simulink model "P2PHVDCMMC"  (R2024a)
settings: Solver=FixedStepDiscrete  StartTime=0.0  StopTime=10  RelTol=1e-3
PreLoadFcn:
  | % HVDCMMCInterconnectionParam
StartFcn:
  | tic
StopFcn:
  | toc
values from neighbouring files (symbols this model uses):
  C_PM = 1.758e-3    (= 0.001758)    [P2PHVDCMMCcode.m]
  Cg = 50e-9    (= 5e-08)    [P2PHVDCMMCcode.m]
  Fc = Fnom*3.37    (= 168.5)    [P2PHVDCMMCcode.m]
  Fnom = 50    [P2PHVDCMMCcode.m]
  Ki_Ireg = 6    [P2PHVDCMMCcode.m]
  Ki_Preg = 1.0    (= 1)    [P2PHVDCMMCcode.m]
  Ki_Qreg = 1.0    (= 1)    [P2PHVDCMMCcode.m]
  Ki_VDCreg = 100    [P2PHVDCMMCcode.m]
  Kp_Ireg = 0.6    [P2PHVDCMMCcode.m]
  Kp_Preg = 0.5/3    (= 0.166666666667)    [P2PHVDCMMCcode.m]
  Kp_Qreg = 0.5/3    (= 0.166666666667)    [P2PHVDCMMCcode.m]
  Kp_VDCreg = 4    [P2PHVDCMMCcode.m]
  L_cable = 15e-3    (= 0.015)    [P2PHVDCMMCcode.m]
  Larm = Larm_pu*(Zb_ac/(2*pi*Fnom))    [P2PHVDCMMCcode.m]
  Larm_pu = 0.15    [P2PHVDCMMCcode.m]
  Lff = Larm_pu/2    (= 0.075)    [P2PHVDCMMCcode.m]
  Limits_Ireg = [ 2.0  -2.0]    [P2PHVDCMMCcode.m]
  Limits_Preg = [ 1.2, 0.8 ]    [P2PHVDCMMCcode.m]
  Limits_Qreg = [ 0.25, -0.25 ]    [P2PHVDCMMCcode.m]
  Limits_VDCreg = [ 2.0  -2.0]    [P2PHVDCMMCcode.m]
  Lxfo = 0.12    [P2PHVDCMMCcode.m]
  N = 1    [P2PHVDCMMCcode.m]
  Nb_PM = 36    [P2PHVDCMMCcode.m]
  Pnom = 1000e6    (= 1000000000)    [P2PHVDCMMCcode.m]
  R_cable = 0.5    [P2PHVDCMMCcode.m]
  R_startup = 400    [P2PHVDCMMCcode.m]
  Rarm = Rarm_pu*Zb_ac    [P2PHVDCMMCcode.m]
  Rff = Rarm_pu/2    (= 0.00075)    [P2PHVDCMMCcode.m]
  Rg = 100    [P2PHVDCMMCcode.m]
  Rxfo = 0.003    [P2PHVDCMMCcode.m]
  Slope_Qref = 0.5    [P2PHVDCMMCcode.m]
  Slope_Vdc_ref = Vnom_dc/5    (= 128000)    [P2PHVDCMMCcode.m]
  Ts = Ts_Control    (= 4e-05)    [P2PHVDCMMCcode.m]
  Ts_Control = 40e-6    (= 4e-05)    [P2PHVDCMMCcode.m]
  Ts_Power = 20e-6    (= 2e-05)    [P2PHVDCMMCcode.m]
  Vnom_dc = 640e3    (= 640000)    [P2PHVDCMMCcode.m]
  Vnom_prim = 400e3    (= 400000)    [P2PHVDCMMCcode.m]
  Vnom_sec = 333e3    (= 333000)    [P2PHVDCMMCcode.m]
undefined symbols (not defined in the file or in its folder): DiscIntNeverNeededParam, Discrete, gcbh, HRM, Pcc, S, sps, sps_rtmsupport, spsMeanValueVariableFrequencyModel, spsPLL3phModel, SY3, Tfault
libraries: simulink x38, spsControlledVoltageSourceLib x30, DQsym_Lib x25, spsVoltageMeasurementLib x21, spsIdealSwitchLib x21, powerlib_extras x12, spsSecondOrderFilterLib x12, spsCurrentMeasurementLib x12, spsdq0toabcLib x9, spsMeanLib x8, spsMeanVariableFrequencyLib x8, spsabctodq0Lib x8
(part 2 of 8)

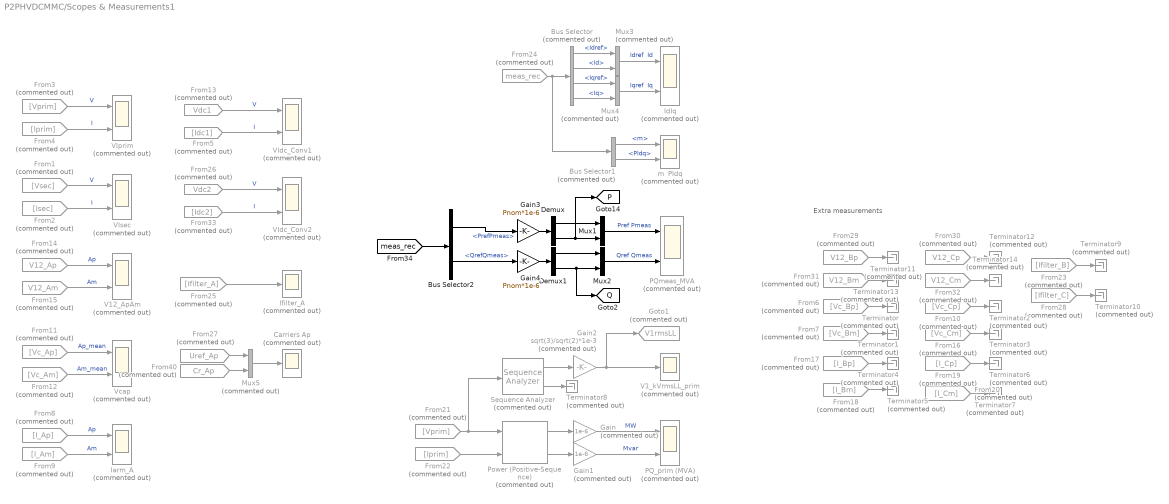
== system P2PHVDCMMC/Scopes & Measurements1 ==
  note: Extra measurements
  Bus Selector : BusSelector  Commented=on  OutputSignals=Idref,Id,Iqref,Iq
  Bus Selector1 : BusSelector  Commented=on  OutputSignals=m,PIdq
  Bus Selector2 : BusSelector  OutputSignals=PrefPmeas,QrefQmeas
  Carriers Ap : Scope  Commented=on
  Demux : Demux  Outputs=2
  Demux1 : Demux  Outputs=2
  From1 : From  Commented=on  GotoTag=Vsec  TagVisibility=global
  From10 : From  Commented=on  GotoTag=Vc_Cp
  From11 : From  Commented=on  GotoTag=Vc_Ap
  From12 : From  Commented=on  GotoTag=Vc_Am
  From13 : From  Commented=on  GotoTag=Vdc1  TagVisibility=global
  From14 : From  Commented=on  GotoTag=V12_Ap
  From15 : From  Commented=on  GotoTag=V12_Am
  From16 : From  Commented=on  GotoTag=Vc_Cm
  From17 : From  Commented=on  GotoTag=I_Bp
  From18 : From  Commented=on  GotoTag=I_Bm
  From19 : From  Commented=on  GotoTag=I_Cp
  From2 : From  Commented=on  GotoTag=Isec  TagVisibility=global
  From20 : From  Commented=on  GotoTag=I_Cm
  From21 : From  Commented=on  GotoTag=Vprim  TagVisibility=global
  From22 : From  Commented=on  GotoTag=Iprim  TagVisibility=global
  From23 : From  Commented=on  GotoTag=Ifilter_B
  From24 : From  Commented=on  GotoTag=meas_rec  TagVisibility=global
  From25 : From  Commented=on  GotoTag=Ifilter_A
  From26 : From  Commented=on  GotoTag=Vdc2  TagVisibility=global
  From27 : From  Commented=on  GotoTag=Uref_Ap  TagVisibility=global
  From28 : From  Commented=on  GotoTag=Ifilter_C
  From29 : From  Commented=on  GotoTag=V12_Bp
  From3 : From  Commented=on  GotoTag=Vprim  TagVisibility=global
  From30 : From  Commented=on  GotoTag=V12_Cp
  From31 : From  Commented=on  GotoTag=V12_Bm
  From32 : From  Commented=on  GotoTag=V12_Cm
  From33 : From  Commented=on  GotoTag=Idc2
  From4 : From  Commented=on  GotoTag=Iprim  TagVisibility=global
  From40 : From  Commented=on  GotoTag=Cr_Ap  TagVisibility=global
  From5 : From  Commented=on  GotoTag=Idc1  TagVisibility=global
  From6 : From  Commented=on  GotoTag=Vc_Bp
  From7 : From  Commented=on  GotoTag=Vc_Bm
  From8 : From  Commented=on  GotoTag=I_Ap
  From9 : From  Commented=on  GotoTag=I_Am
  Gain : Gain  Commented=on  Gain=1e-6
  Gain1 : Gain  Commented=on  Gain=1e-6
  Gain2 : Gain  Commented=on  Gain=sqrt(3)/sqrt(2)*1e-3
  Gain3 : Gain  Gain=Pnom*1e-6
  Gain4 : Gain  Gain=Pnom*1e-6
  Goto1 : Goto  Commented=on  GotoTag=V1rmsLL  TagVisibility=global
  Iarm_A : Scope  Commented=on  NumInputPorts=2
  IdIq : Scope  Commented=on  NumInputPorts=2
  Ifilter_A : Scope  Commented=on
  Mux1 : Mux  Inputs=2
  Mux2 : Mux  Inputs=2
  Mux3 : Mux  Commented=on  Inputs=2
  Mux4 : Mux  Commented=on  Inputs=2
  Mux5 : Mux  Commented=on  Inputs=2
  PQ_prim (MVA) : Scope  Commented=on  NumInputPorts=2
  PQmeas_MVA : Scope  Commented=on  NumInputPorts=2
  Power (Positive-Sequence) : spsPowerPositiveSequenceLib/Power (Positive-Sequence)  Commented=on  Freq=Fnom  Vinit=[0, 0]  Iinit=[0, 0]  Ts=Ts_Power
  Sequence Analyzer : spsSequenceAnalyzerLib/Sequence Analyzer  Commented=on  Freq=Fnom  n=1  seq=Positive  InInit=[1, 0]  Ts=Ts_Power
  Terminator{,1..14} (15 alike) : Terminator  Commented=on
  V12_ApAm : Scope  Commented=on  NumInputPorts=2
  V1_kVrmsLL_prim : Scope  Commented=on
  VIdc_Conv1 : Scope  Commented=on  NumInputPorts=2
  VIdc_Conv2 : Scope  Commented=on  NumInputPorts=2
  VIprim : Scope  Commented=on  NumInputPorts=2
  VIsec : Scope  Commented=on  NumInputPorts=2
  Vcap : Scope  Commented=on  NumInputPorts=2
  m  PIdq : Scope  Commented=on  NumInputPorts=2
  tag scope: P=global, Q=global
  wires:
  Mux5/1 -> Carriers Ap/1
  From40/1 -> Mux5/2
  From27/1 -> Mux5/1
  From12/1 -> Vcap/2  "Am_mean"
  From11/1 -> Vcap/1  "Ap_mean"
  From33/1 -> VIdc_Conv2/2  "I"
  From26/1 -> VIdc_Conv2/1  "V"
  Gain4/1 -> Demux1/1
  Gain3/1 -> Demux/1
  Mux2/1 -> PQmeas_MVA/2  "Qref Qmeas"
  Bus Selector2/2 -> Gain4/1  "<QrefQmeas>"
  Bus Selector2/1 -> Gain3/1  "<PrefPmeas>"
  Mux1/1 -> PQmeas_MVA/1  "Pref Pmeas"
  [meas_rec] -> Bus Selector2/1
  Gain2/1 -> V1_kVrmsLL_prim/1, Goto1/1
  Gain1/1 -> PQ_prim (MVA)/2  "Mvar"
  Gain/1 -> PQ_prim (MVA)/1  "MW"
  From32/1 -> Terminator14/1
  From31/1 -> Terminator13/1
  From30/1 -> Terminator12/1
  From29/1 -> Terminator11/1
  From28/1 -> Terminator10/1
  From23/1 -> Terminator9/1
  Sequence Analyzer/1 -> Gain2/1
  Power (Positive-Sequence)/2 -> Gain1/1
  Power (Positive-Sequence)/1 -> Gain/1
  Sequence Analyzer/2 -> Terminator8/1
  From22/1 -> Power (Positive-Sequence)/2
  From21/1 -> Power (Positive-Sequence)/1, Sequence Analyzer/1
  From5/1 -> VIdc_Conv1/2  "I"
  From13/1 -> VIdc_Conv1/1  "V"
  From25/1 -> Ifilter_A/1
  Bus Selector/4 -> Mux4/2  "<Iq>"
  Bus Selector/3 -> Mux4/1  "<Iqref>"
  Bus Selector/2 -> Mux3/2  "<Id>"
  Bus Selector/1 -> Mux3/1  "<Idref>"
  Mux4/1 -> IdIq/2  "Iqref  Iq"
  Mux3/1 -> IdIq/1  "Idref  Id"
  Bus Selector1/2 -> m  PIdq/2  "<PIdq>"
  Bus Selector1/1 -> m  PIdq/1  "<m>"
  From24/1 -> Bus Selector/1, Bus Selector1/1
  From20/1 -> Terminator7/1
  From19/1 -> Terminator6/1
  From18/1 -> Terminator5/1
  From17/1 -> Terminator4/1
  From9/1 -> Iarm_A/2  "Am"
  From8/1 -> Iarm_A/1  "Ap"
  From16/1 -> Terminator3/1
  From10/1 -> Terminator2/1
  From7/1 -> Terminator1/1
  From6/1 -> Terminator/1
  From15/1 -> V12_ApAm/2  "Am"
  From14/1 -> V12_ApAm/1  "Ap"
  From1/1 -> VIsec/1  "V"
  From2/1 -> VIsec/2  "I"
  From3/1 -> VIprim/1  "V"
  From4/1 -> VIprim/2  "I"
  Demux/1 -> Mux1/1
  Demux/2 -> [P], Mux1/2
  Demux1/1 -> Mux2/1
  Demux1/2 -> [Q], Mux2/2

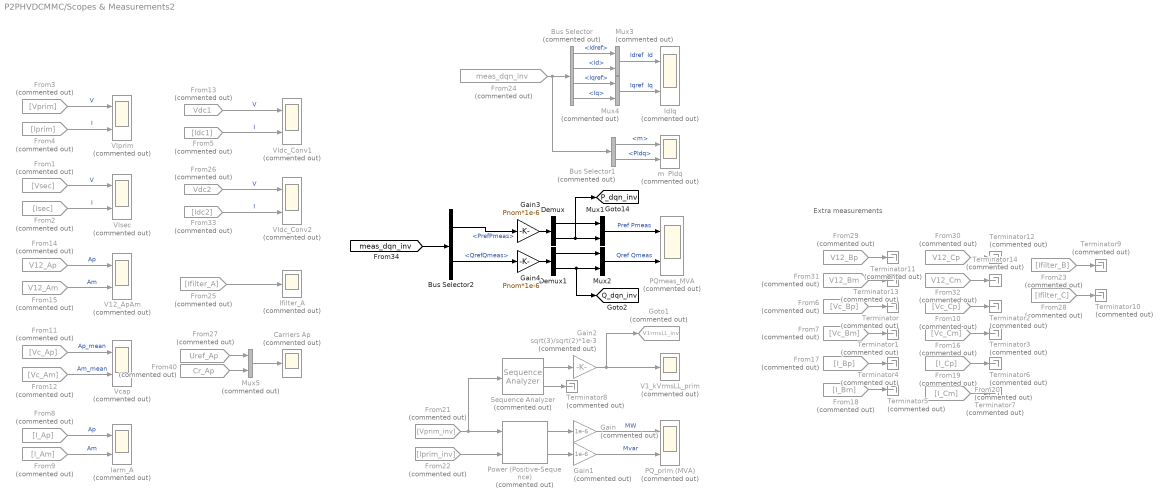
== system P2PHVDCMMC/Scopes & Measurements2 ==
  note: Extra measurements
  Bus Selector : BusSelector  Commented=on  OutputSignals=Idref,Id,Iqref,Iq
  Bus Selector1 : BusSelector  Commented=on  OutputSignals=m,PIdq
  Bus Selector2 : BusSelector  OutputSignals=PrefPmeas,QrefQmeas
  Carriers Ap : Scope  Commented=on
  Demux : Demux  Outputs=2
  Demux1 : Demux  Outputs=2
  From1 : From  Commented=on  GotoTag=Vsec  TagVisibility=global
  From10 : From  Commented=on  GotoTag=Vc_Cp
  From11 : From  Commented=on  GotoTag=Vc_Ap
  From12 : From  Commented=on  GotoTag=Vc_Am
  From13 : From  Commented=on  GotoTag=Vdc1  TagVisibility=global
  From14 : From  Commented=on  GotoTag=V12_Ap
  From15 : From  Commented=on  GotoTag=V12_Am
  From16 : From  Commented=on  GotoTag=Vc_Cm
  From17 : From  Commented=on  GotoTag=I_Bp
  From18 : From  Commented=on  GotoTag=I_Bm
  From19 : From  Commented=on  GotoTag=I_Cp
  From2 : From  Commented=on  GotoTag=Isec  TagVisibility=global
  From20 : From  Commented=on  GotoTag=I_Cm
  From21 : From  Commented=on  GotoTag=Vprim_inv  TagVisibility=global
  From22 : From  Commented=on  GotoTag=Iprim_inv  TagVisibility=global
  From23 : From  Commented=on  GotoTag=Ifilter_B
  From24 : From  Commented=on  GotoTag=meas_dqn_inv  TagVisibility=global
  From25 : From  Commented=on  GotoTag=Ifilter_A
  From26 : From  Commented=on  GotoTag=Vdc2  TagVisibility=global
  From27 : From  Commented=on  GotoTag=Uref_Ap  TagVisibility=global
  From28 : From  Commented=on  GotoTag=Ifilter_C
  From29 : From  Commented=on  GotoTag=V12_Bp
  From3 : From  Commented=on  GotoTag=Vprim  TagVisibility=global
  From30 : From  Commented=on  GotoTag=V12_Cp
  From31 : From  Commented=on  GotoTag=V12_Bm
  From32 : From  Commented=on  GotoTag=V12_Cm
  From33 : From  Commented=on  GotoTag=Idc2  TagVisibility=global
  From4 : From  Commented=on  GotoTag=Iprim  TagVisibility=global
  From40 : From  Commented=on  GotoTag=Cr_Ap  TagVisibility=global
  From5 : From  Commented=on  GotoTag=Idc1  TagVisibility=global
  From6 : From  Commented=on  GotoTag=Vc_Bp
  From7 : From  Commented=on  GotoTag=Vc_Bm
  From8 : From  Commented=on  GotoTag=I_Ap
  From9 : From  Commented=on  GotoTag=I_Am
  Gain : Gain  Commented=on  Gain=1e-6
  Gain1 : Gain  Commented=on  Gain=1e-6
  Gain2 : Gain  Commented=on  Gain=sqrt(3)/sqrt(2)*1e-3
  Gain3 : Gain  Gain=Pnom*1e-6
  Gain4 : Gain  Gain=Pnom*1e-6
  Goto1 : Goto  Commented=on  GotoTag=V1rmsLL_inv  TagVisibility=global
  Iarm_A : Scope  Commented=on  NumInputPorts=2
  IdIq : Scope  Commented=on  NumInputPorts=2
  Ifilter_A : Scope  Commented=on
  Mux1 : Mux  Inputs=2
  Mux2 : Mux  Inputs=2
  Mux3 : Mux  Commented=on  Inputs=2
  Mux4 : Mux  Commented=on  Inputs=2
  Mux5 : Mux  Commented=on  Inputs=2
  PQ_prim (MVA) : Scope  Commented=on  NumInputPorts=2
  PQmeas_MVA : Scope  Commented=on  NumInputPorts=2
  Power (Positive-Sequence) : spsPowerPositiveSequenceLib/Power (Positive-Sequence)  Commented=on  Freq=Fnom  Vinit=[0, 0]  Iinit=[0, 0]  Ts=Ts_Power
  Sequence Analyzer : spsSequenceAnalyzerLib/Sequence Analyzer  Commented=on  Freq=Fnom  n=1  seq=Positive  InInit=[1, 0]  Ts=Ts_Power
  Terminator{,1..14} (15 alike) : Terminator  Commented=on
  V12_ApAm : Scope  Commented=on  NumInputPorts=2
  V1_kVrmsLL_prim : Scope  Commented=on
  VIdc_Conv1 : Scope  Commented=on  NumInputPorts=2
  VIdc_Conv2 : Scope  Commented=on  NumInputPorts=2
  VIprim : Scope  Commented=on  NumInputPorts=2
  VIsec : Scope  Commented=on  NumInputPorts=2
  Vcap : Scope  Commented=on  NumInputPorts=2
  m  PIdq : Scope  Commented=on  NumInputPorts=2
  tag scope: P_dqn_inv=global, Q_dqn_inv=global
  wires:
  Demux1/2 -> Mux2/2, [Q_dqn_inv]
  Demux1/1 -> Mux2/1
  Demux/2 -> Mux1/2, [P_dqn_inv]
  Demux/1 -> Mux1/1
  From4/1 -> VIprim/2  "I"
  From3/1 -> VIprim/1  "V"
  From2/1 -> VIsec/2  "I"
  From1/1 -> VIsec/1  "V"
  From14/1 -> V12_ApAm/1  "Ap"
  From15/1 -> V12_ApAm/2  "Am"
  From6/1 -> Terminator/1
  From7/1 -> Terminator1/1
  From10/1 -> Terminator2/1
  From16/1 -> Terminator3/1
  From8/1 -> Iarm_A/1  "Ap"
  From9/1 -> Iarm_A/2  "Am"
  From17/1 -> Terminator4/1
  From18/1 -> Terminator5/1
  From19/1 -> Terminator6/1
  From20/1 -> Terminator7/1
  From24/1 -> Bus Selector1/1, Bus Selector/1
  Bus Selector1/1 -> m  PIdq/1  "<m>"
  Bus Selector1/2 -> m  PIdq/2  "<PIdq>"
  Mux3/1 -> IdIq/1  "Idref  Id"
  Mux4/1 -> IdIq/2  "Iqref  Iq"
  Bus Selector/1 -> Mux3/1  "<Idref>"
  Bus Selector/2 -> Mux3/2  "<Id>"
  Bus Selector/3 -> Mux4/1  "<Iqref>"
  Bus Selector/4 -> Mux4/2  "<Iq>"
  From25/1 -> Ifilter_A/1
  From13/1 -> VIdc_Conv1/1  "V"
  From5/1 -> VIdc_Conv1/2  "I"
  From21/1 -> Sequence Analyzer/1, Power (Positive-Sequence)/1
  From22/1 -> Power (Positive-Sequence)/2
  Sequence Analyzer/2 -> Terminator8/1
  Power (Positive-Sequence)/1 -> Gain/1
  Power (Positive-Sequence)/2 -> Gain1/1
  Sequence Analyzer/1 -> Gain2/1
  From23/1 -> Terminator9/1
  From28/1 -> Terminator10/1
  From29/1 -> Terminator11/1
  From30/1 -> Terminator12/1
  From31/1 -> Terminator13/1
  From32/1 -> Terminator14/1
  Gain/1 -> PQ_prim (MVA)/1  "MW"
  Gain1/1 -> PQ_prim (MVA)/2  "Mvar"
  Gain2/1 -> Goto1/1, V1_kVrmsLL_prim/1
  [meas_dqn_inv] -> Bus Selector2/1
  Mux1/1 -> PQmeas_MVA/1  "Pref Pmeas"
  Bus Selector2/1 -> Gain3/1  "<PrefPmeas>"
  Bus Selector2/2 -> Gain4/1  "<QrefQmeas>"
  Mux2/1 -> PQmeas_MVA/2  "Qref Qmeas"
  Gain3/1 -> Demux/1
  Gain4/1 -> Demux1/1
  From26/1 -> VIdc_Conv2/1  "V"
  From33/1 -> VIdc_Conv2/2  "I"
  From11/1 -> Vcap/1  "Ap_mean"
  From12/1 -> Vcap/2  "Am_mean"
  From27/1 -> Mux5/1
  From40/1 -> Mux5/2
  Mux5/1 -> Carriers Ap/1

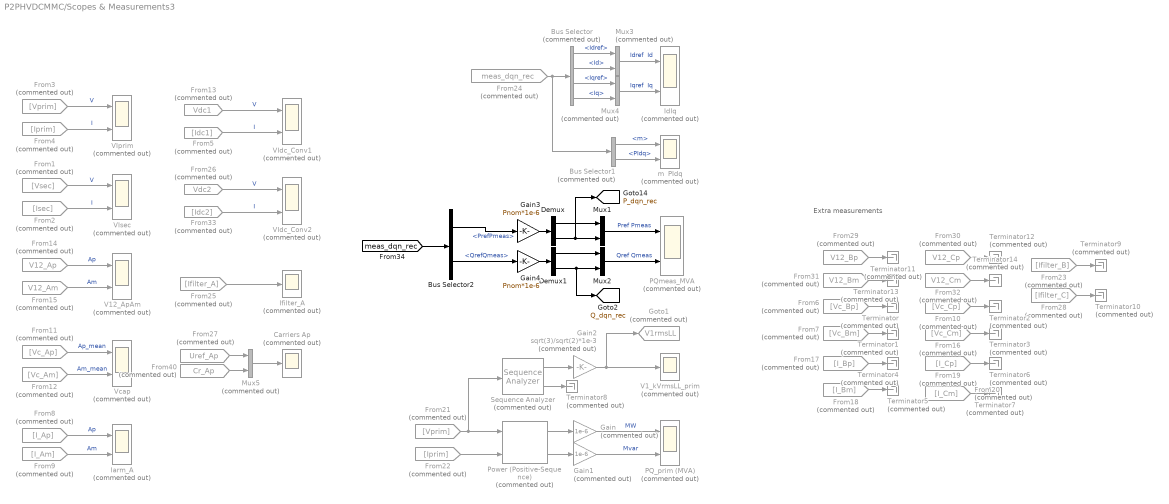
== system P2PHVDCMMC/Scopes & Measurements3 ==
  note: Extra measurements
  Bus Selector : BusSelector  Commented=on  OutputSignals=Idref,Id,Iqref,Iq
  Bus Selector1 : BusSelector  Commented=on  OutputSignals=m,PIdq
  Bus Selector2 : BusSelector  OutputSignals=PrefPmeas,QrefQmeas
  Carriers Ap : Scope  Commented=on
  Demux : Demux  Outputs=2
  Demux1 : Demux  Outputs=2
  From1 : From  Commented=on  GotoTag=Vsec  TagVisibility=global
  From10 : From  Commented=on  GotoTag=Vc_Cp
  From11 : From  Commented=on  GotoTag=Vc_Ap
  From12 : From  Commented=on  GotoTag=Vc_Am
  From13 : From  Commented=on  GotoTag=Vdc1  TagVisibility=global
  From14 : From  Commented=on  GotoTag=V12_Ap
  From15 : From  Commented=on  GotoTag=V12_Am
  From16 : From  Commented=on  GotoTag=Vc_Cm
  From17 : From  Commented=on  GotoTag=I_Bp
  From18 : From  Commented=on  GotoTag=I_Bm
  From19 : From  Commented=on  GotoTag=I_Cp
  From2 : From  Commented=on  GotoTag=Isec  TagVisibility=global
  From20 : From  Commented=on  GotoTag=I_Cm
  From21 : From  Commented=on  GotoTag=Vprim  TagVisibility=global
  From22 : From  Commented=on  GotoTag=Iprim  TagVisibility=global
  From23 : From  Commented=on  GotoTag=Ifilter_B
  From24 : From  Commented=on  GotoTag=meas_dqn_rec  TagVisibility=global
  From25 : From  Commented=on  GotoTag=Ifilter_A
  From26 : From  Commented=on  GotoTag=Vdc2  TagVisibility=global
  From27 : From  Commented=on  GotoTag=Uref_Ap  TagVisibility=global
  From28 : From  Commented=on  GotoTag=Ifilter_C
  From29 : From  Commented=on  GotoTag=V12_Bp
  From3 : From  Commented=on  GotoTag=Vprim  TagVisibility=global
  From30 : From  Commented=on  GotoTag=V12_Cp
  From31 : From  Commented=on  GotoTag=V12_Bm
  From32 : From  Commented=on  GotoTag=V12_Cm
  From33 : From  Commented=on  GotoTag=Idc2  TagVisibility=global
  From4 : From  Commented=on  GotoTag=Iprim  TagVisibility=global
  From40 : From  Commented=on  GotoTag=Cr_Ap  TagVisibility=global
  From5 : From  Commented=on  GotoTag=Idc1  TagVisibility=global
  From6 : From  Commented=on  GotoTag=Vc_Bp
  From7 : From  Commented=on  GotoTag=Vc_Bm
  From8 : From  Commented=on  GotoTag=I_Ap
  From9 : From  Commented=on  GotoTag=I_Am
  Gain : Gain  Commented=on  Gain=1e-6
  Gain1 : Gain  Commented=on  Gain=1e-6
  Gain2 : Gain  Commented=on  Gain=sqrt(3)/sqrt(2)*1e-3
  Gain3 : Gain  Gain=Pnom*1e-6
  Gain4 : Gain  Gain=Pnom*1e-6
  Goto1 : Goto  Commented=on  GotoTag=V1rmsLL  TagVisibility=global
  Iarm_A : Scope  Commented=on  NumInputPorts=2
  IdIq : Scope  Commented=on  NumInputPorts=2
  Ifilter_A : Scope  Commented=on
  Mux1 : Mux  Inputs=2
  Mux2 : Mux  Inputs=2
  Mux3 : Mux  Commented=on  Inputs=2
  Mux4 : Mux  Commented=on  Inputs=2
  Mux5 : Mux  Commented=on  Inputs=2
  PQ_prim (MVA) : Scope  Commented=on  NumInputPorts=2
  PQmeas_MVA : Scope  Commented=on  NumInputPorts=2
  Power (Positive-Sequence) : spsPowerPositiveSequenceLib/Power (Positive-Sequence)  Commented=on  Freq=Fnom  Vinit=[0, 0]  Iinit=[0, 0]  Ts=Ts_Power
  Sequence Analyzer : spsSequenceAnalyzerLib/Sequence Analyzer  Commented=on  Freq=Fnom  n=1  seq=Positive  InInit=[1, 0]  Ts=Ts_Power
  Terminator{,1..14} (15 alike) : Terminator  Commented=on
  V12_ApAm : Scope  Commented=on  NumInputPorts=2
  V1_kVrmsLL_prim : Scope  Commented=on
  VIdc_Conv1 : Scope  Commented=on  NumInputPorts=2
  VIdc_Conv2 : Scope  Commented=on  NumInputPorts=2
  VIprim : Scope  Commented=on  NumInputPorts=2
  VIsec : Scope  Commented=on  NumInputPorts=2
  Vcap : Scope  Commented=on  NumInputPorts=2
  m  PIdq : Scope  Commented=on  NumInputPorts=2
  tag scope: P_dqn_rec=global, Q_dqn_rec=global
  wires:
  Demux1/2 -> Mux2/2, [Q_dqn_rec]
  Demux1/1 -> Mux2/1
  Demux/2 -> Mux1/2, [P_dqn_rec]
  Demux/1 -> Mux1/1
  From4/1 -> VIprim/2  "I"
  From3/1 -> VIprim/1  "V"
  From2/1 -> VIsec/2  "I"
  From1/1 -> VIsec/1  "V"
  From14/1 -> V12_ApAm/1  "Ap"
  From15/1 -> V12_ApAm/2  "Am"
  From6/1 -> Terminator/1
  From7/1 -> Terminator1/1
  From10/1 -> Terminator2/1
  From16/1 -> Terminator3/1
  From8/1 -> Iarm_A/1  "Ap"
  From9/1 -> Iarm_A/2  "Am"
  From17/1 -> Terminator4/1
  From18/1 -> Terminator5/1
  From19/1 -> Terminator6/1
  From20/1 -> Terminator7/1
  From24/1 -> Bus Selector1/1, Bus Selector/1
  Bus Selector1/1 -> m  PIdq/1  "<m>"
  Bus Selector1/2 -> m  PIdq/2  "<PIdq>"
  Mux3/1 -> IdIq/1  "Idref  Id"
  Mux4/1 -> IdIq/2  "Iqref  Iq"
  Bus Selector/1 -> Mux3/1  "<Idref>"
  Bus Selector/2 -> Mux3/2  "<Id>"
  Bus Selector/3 -> Mux4/1  "<Iqref>"
  Bus Selector/4 -> Mux4/2  "<Iq>"
  From25/1 -> Ifilter_A/1
  From13/1 -> VIdc_Conv1/1  "V"
  From5/1 -> VIdc_Conv1/2  "I"
  From21/1 -> Sequence Analyzer/1, Power (Positive-Sequence)/1
  From22/1 -> Power (Positive-Sequence)/2
  Sequence Analyzer/2 -> Terminator8/1
  Power (Positive-Sequence)/1 -> Gain/1
  Power (Positive-Sequence)/2 -> Gain1/1
  Sequence Analyzer/1 -> Gain2/1
  From23/1 -> Terminator9/1
  From28/1 -> Terminator10/1
  From29/1 -> Terminator11/1
  From30/1 -> Terminator12/1
  From31/1 -> Terminator13/1
  From32/1 -> Terminator14/1
  Gain/1 -> PQ_prim (MVA)/1  "MW"
  Gain1/1 -> PQ_prim (MVA)/2  "Mvar"
  Gain2/1 -> Goto1/1, V1_kVrmsLL_prim/1
  [meas_dqn_rec] -> Bus Selector2/1
  Mux1/1 -> PQmeas_MVA/1  "Pref Pmeas"
  Bus Selector2/1 -> Gain3/1  "<PrefPmeas>"
  Bus Selector2/2 -> Gain4/1  "<QrefQmeas>"
  Mux2/1 -> PQmeas_MVA/2  "Qref Qmeas"
  Gain3/1 -> Demux/1
  Gain4/1 -> Demux1/1
  From26/1 -> VIdc_Conv2/1  "V"
  From33/1 -> VIdc_Conv2/2  "I"
  From11/1 -> Vcap/1  "Ap_mean"
  From12/1 -> Vcap/2  "Am_mean"
  From27/1 -> Mux5/1
  From40/1 -> Mux5/2
  Mux5/1 -> Carriers Ap/1

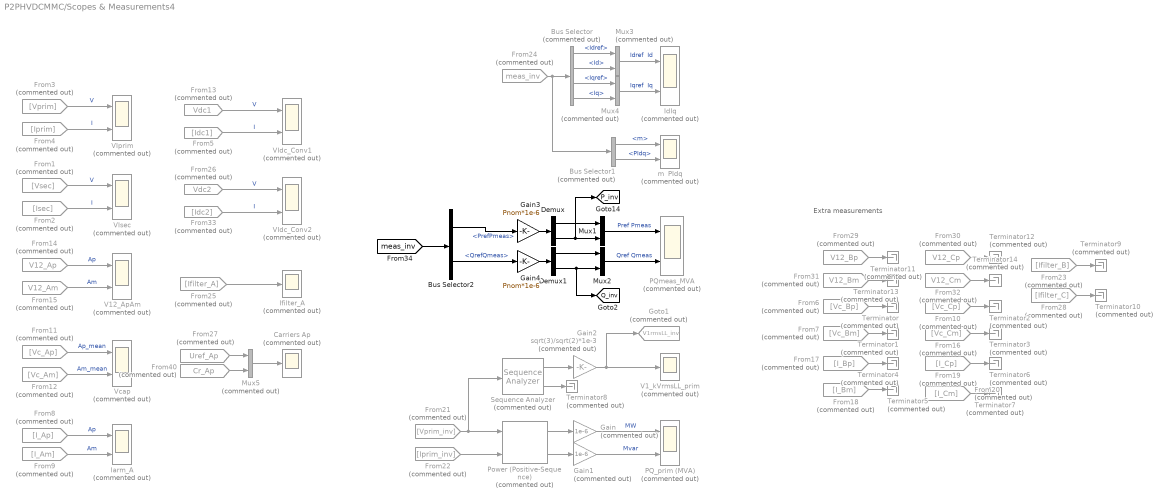
== system P2PHVDCMMC/Scopes & Measurements4 ==
  note: Extra measurements
  Bus Selector : BusSelector  Commented=on  OutputSignals=Idref,Id,Iqref,Iq
  Bus Selector1 : BusSelector  Commented=on  OutputSignals=m,PIdq
  Bus Selector2 : BusSelector  OutputSignals=PrefPmeas,QrefQmeas
  Carriers Ap : Scope  Commented=on
  Demux : Demux  Outputs=2
  Demux1 : Demux  Outputs=2
  From1 : From  Commented=on  GotoTag=Vsec  TagVisibility=global
  From10 : From  Commented=on  GotoTag=Vc_Cp
  From11 : From  Commented=on  GotoTag=Vc_Ap
  From12 : From  Commented=on  GotoTag=Vc_Am
  From13 : From  Commented=on  GotoTag=Vdc1  TagVisibility=global
  From14 : From  Commented=on  GotoTag=V12_Ap
  From15 : From  Commented=on  GotoTag=V12_Am
  From16 : From  Commented=on  GotoTag=Vc_Cm
  From17 : From  Commented=on  GotoTag=I_Bp
  From18 : From  Commented=on  GotoTag=I_Bm
  From19 : From  Commented=on  GotoTag=I_Cp
  From2 : From  Commented=on  GotoTag=Isec  TagVisibility=global
  From20 : From  Commented=on  GotoTag=I_Cm
  From21 : From  Commented=on  GotoTag=Vprim_inv  TagVisibility=global
  From22 : From  Commented=on  GotoTag=Iprim_inv  TagVisibility=global
  From23 : From  Commented=on  GotoTag=Ifilter_B
  From24 : From  Commented=on  GotoTag=meas_inv  TagVisibility=global
  From25 : From  Commented=on  GotoTag=Ifilter_A
  From26 : From  Commented=on  GotoTag=Vdc2  TagVisibility=global
  From27 : From  Commented=on  GotoTag=Uref_Ap  TagVisibility=global
  From28 : From  Commented=on  GotoTag=Ifilter_C
  From29 : From  Commented=on  GotoTag=V12_Bp
  From3 : From  Commented=on  GotoTag=Vprim  TagVisibility=global
  From30 : From  Commented=on  GotoTag=V12_Cp
  From31 : From  Commented=on  GotoTag=V12_Bm
  From32 : From  Commented=on  GotoTag=V12_Cm
  From33 : From  Commented=on  GotoTag=Idc2  TagVisibility=global
  From4 : From  Commented=on  GotoTag=Iprim  TagVisibility=global
  From40 : From  Commented=on  GotoTag=Cr_Ap  TagVisibility=global
  From5 : From  Commented=on  GotoTag=Idc1  TagVisibility=global
  From6 : From  Commented=on  GotoTag=Vc_Bp
  From7 : From  Commented=on  GotoTag=Vc_Bm
  From8 : From  Commented=on  GotoTag=I_Ap
  From9 : From  Commented=on  GotoTag=I_Am
  Gain : Gain  Commented=on  Gain=1e-6
  Gain1 : Gain  Commented=on  Gain=1e-6
  Gain2 : Gain  Commented=on  Gain=sqrt(3)/sqrt(2)*1e-3
  Gain3 : Gain  Gain=Pnom*1e-6
  Gain4 : Gain  Gain=Pnom*1e-6
  Goto1 : Goto  Commented=on  GotoTag=V1rmsLL_inv  TagVisibility=global
  Iarm_A : Scope  Commented=on  NumInputPorts=2
  IdIq : Scope  Commented=on  NumInputPorts=2
  Ifilter_A : Scope  Commented=on
  Mux1 : Mux  Inputs=2
  Mux2 : Mux  Inputs=2
  Mux3 : Mux  Commented=on  Inputs=2
  Mux4 : Mux  Commented=on  Inputs=2
  Mux5 : Mux  Commented=on  Inputs=2
  PQ_prim (MVA) : Scope  Commented=on  NumInputPorts=2
  PQmeas_MVA : Scope  Commented=on  NumInputPorts=2
  Power (Positive-Sequence) : spsPowerPositiveSequenceLib/Power (Positive-Sequence)  Commented=on  Freq=Fnom  Vinit=[0, 0]  Iinit=[0, 0]  Ts=Ts_Power
  Sequence Analyzer : spsSequenceAnalyzerLib/Sequence Analyzer  Commented=on  Freq=Fnom  n=1  seq=Positive  InInit=[1, 0]  Ts=Ts_Power
  Terminator{,1..14} (15 alike) : Terminator  Commented=on
  V12_ApAm : Scope  Commented=on  NumInputPorts=2
  V1_kVrmsLL_prim : Scope  Commented=on
  VIdc_Conv1 : Scope  Commented=on  NumInputPorts=2
  VIdc_Conv2 : Scope  Commented=on  NumInputPorts=2
  VIprim : Scope  Commented=on  NumInputPorts=2
  VIsec : Scope  Commented=on  NumInputPorts=2
  Vcap : Scope  Commented=on  NumInputPorts=2
  m  PIdq : Scope  Commented=on  NumInputPorts=2
  tag scope: P_inv=global, Q_inv=global
  wires:
  Mux5/1 -> Carriers Ap/1
  From40/1 -> Mux5/2
  From27/1 -> Mux5/1
  From12/1 -> Vcap/2  "Am_mean"
  From11/1 -> Vcap/1  "Ap_mean"
  From33/1 -> VIdc_Conv2/2  "I"
  From26/1 -> VIdc_Conv2/1  "V"
  Gain4/1 -> Demux1/1
  Gain3/1 -> Demux/1
  Mux2/1 -> PQmeas_MVA/2  "Qref Qmeas"
  Bus Selector2/2 -> Gain4/1  "<QrefQmeas>"
  Bus Selector2/1 -> Gain3/1  "<PrefPmeas>"
  Mux1/1 -> PQmeas_MVA/1  "Pref Pmeas"
  [meas_inv] -> Bus Selector2/1
  Gain2/1 -> V1_kVrmsLL_prim/1, Goto1/1
  Gain1/1 -> PQ_prim (MVA)/2  "Mvar"
  Gain/1 -> PQ_prim (MVA)/1  "MW"
  From32/1 -> Terminator14/1
  From31/1 -> Terminator13/1
  From30/1 -> Terminator12/1
  From29/1 -> Terminator11/1
  From28/1 -> Terminator10/1
  From23/1 -> Terminator9/1
  Sequence Analyzer/1 -> Gain2/1
  Power (Positive-Sequence)/2 -> Gain1/1
  Power (Positive-Sequence)/1 -> Gain/1
  Sequence Analyzer/2 -> Terminator8/1
  From22/1 -> Power (Positive-Sequence)/2
  From21/1 -> Power (Positive-Sequence)/1, Sequence Analyzer/1
  From5/1 -> VIdc_Conv1/2  "I"
  From13/1 -> VIdc_Conv1/1  "V"
  From25/1 -> Ifilter_A/1
  Bus Selector/4 -> Mux4/2  "<Iq>"
  Bus Selector/3 -> Mux4/1  "<Iqref>"
  Bus Selector/2 -> Mux3/2  "<Id>"
  Bus Selector/1 -> Mux3/1  "<Idref>"
  Mux4/1 -> IdIq/2  "Iqref  Iq"
  Mux3/1 -> IdIq/1  "Idref  Id"
  Bus Selector1/2 -> m  PIdq/2  "<PIdq>"
  Bus Selector1/1 -> m  PIdq/1  "<m>"
  From24/1 -> Bus Selector/1, Bus Selector1/1
  From20/1 -> Terminator7/1
  From19/1 -> Terminator6/1
  From18/1 -> Terminator5/1
  From17/1 -> Terminator4/1
  From9/1 -> Iarm_A/2  "Am"
  From8/1 -> Iarm_A/1  "Ap"
  From16/1 -> Terminator3/1
  From10/1 -> Terminator2/1
  From7/1 -> Terminator1/1
  From6/1 -> Terminator/1
  From15/1 -> V12_ApAm/2  "Am"
  From14/1 -> V12_ApAm/1  "Ap"
  From1/1 -> VIsec/1  "V"
  From2/1 -> VIsec/2  "I"
  From3/1 -> VIprim/1  "V"
  From4/1 -> VIprim/2  "I"
  Demux/1 -> Mux1/1
  Demux/2 -> [P_inv], Mux1/2
  Demux1/1 -> Mux2/1
  Demux1/2 -> [Q_inv], Mux2/2

== system P2PHVDCMMC/Sequencer2 ==
  note: STEP 2 : Deblocking converter 1
  note: STEP 6: Reactive power regulator setpoint
  note: STEP 1 : Energization
  note: Block the converter when a fault occur
  note: STEP 5: Active power regulator setpoint
  note: STEP 3 : Voltage regulator setpoint
  note: STEP 4: Enable PQ regulators and converter 2
  note: Block the converter when a fault occur
  note: Open breaker 1 when a fault occur
  BL1 : Step  Time=0.07  SampleTime=Ts
  BL12 : Step  Time=Tfault+Ts_Power  SampleTime=Ts_Power
  BL13 : Step  Time=0.05  SampleTime=Ts_Power
  BL14 : Step  Time=0  SampleTime=Ts_Power
  BL15 : Step  Commented=on  Time=0.1  SampleTime=Ts
  BL16 : Step  Time=0.07  Before=1  After=0  SampleTime=Ts_Power
  BL17 : Step  Time=0.07  SampleTime=Ts
  BL18 : Step  Time=Tfault + 1.95*(1/Fnom)  Before=1  After=0  SampleTime=Ts_Power
  BL19 : Step  Time=Tfault + 2*(1/Fnom)  Before=1  After=0  SampleTime=Ts_Power
  BL20 : Step  Time=0.15  SampleTime=Ts_Power
  Constant10 : Constant  Value=-0.35
  Constant2 : Constant  Value=0.5
  Constant3 : Constant  Value=0
  Constant6 : Constant  Value=0.99
  Constant8 : Constant  Value=0.2
  Constant9 : Constant  Value=.8
  Goto11 : Goto  Commented=on  GotoTag=Vdc_ref  TagVisibility=global
  Logical Operator3 : Logic  AllPortsSameDT=off  OutDataTypeStr=boolean
  Logical Operator4 : Logic  Operator=OR  AllPortsSameDT=off  OutDataTypeStr=float('double')
  Logical Operator5 : Logic  AllPortsSameDT=off  OutDataTypeStr=boolean
  Qref2 : simulink/Sources/Ramp  Commented=on  slope=Slope_Qref  start=Tramping_Qref  InitialOutput=0
  Rate Transition1 : RateTransition  OutPortSampleTime=Ts_Control
  Rate Transition2 : RateTransition  OutPortSampleTime=Ts_Control
  Rate Transition6 : RateTransition  Commented=on  OutPortSampleTime=Ts_Control
  Saturation3 : Saturate  Commented=on  UpperLimit=Vnom_dc  LowerLimit=eps
  Saturation4 : Saturate  UpperLimit=1  LowerLimit=-1
  Saturation5 : Saturate  UpperLimit=Limits_Qreg(1)  LowerLimit=Limits_Qreg(2)
  Scope : Scope  Commented=on  NumInputPorts=2
  Step1 : Step  Time=4  Before=1  After=0  SampleTime=0
  Step4 : Step  Time=3  Before=1  After=0  SampleTime=0
  Step5 : Step  Time=6  Before=1  After=0  SampleTime=0
  Step6 : Step  Time=8  Before=1  After=0  SampleTime=0
  Switch{1,4..6} (4 alike) : Switch  Criteria=u2 > Threshold  SaturateOnIntegerOverflow=off  InputSameDT=off
  Vdc_ref 2 : simulink/Sources/Ramp  Commented=on  slope=Slope_Vdc_ref  start=Tramping_Vdc_ref  InitialOutput=Vnom_sec*1.37
  tag scope: Blk=global, Brk1_On=global, Brk2_On=global, Converter2_On=global, PQreg_On=global, Pref=global, Qref=global, VDCreg_On=global
  wires:
  Constant2/1 -> Switch6/3
  Logical Operator5/1 -> [Converter2_On]
  BL20/1 -> Logical Operator3/1
  Switch6/1 -> Scope/1, Saturation4/1
  Switch5/1 -> Switch6/1
  BL14/1 -> Logical Operator5/1
  Constant3/1 -> Saturation5/1, Scope/2, Switch4/1
  Saturation4/1 -> Rate Transition1/1
  Logical Operator4/1 -> [Blk]
  Switch1/1 -> Switch5/1
  Vdc_ref 2/1 -> Saturation3/1
  Saturation5/1 -> Rate Transition2/1
  BL17/1 -> [PQreg_On]
  BL1/1 -> [VDCreg_On]
  BL18/1 -> Logical Operator3/2
  Logical Operator3/1 -> [Brk1_On]
  Constant6/1 -> Switch1/1
  BL16/1 -> Logical Operator4/1
  BL12/1 -> Logical Operator4/2
  Rate Transition6/1 -> Goto11/1
  Rate Transition1/1 -> [Pref]
  Rate Transition2/1 -> [Qref]
  Step1/1 -> Switch1/2
  Constant9/1 -> Switch4/3
  Step4/1 -> Switch4/2
  Constant8/1 -> Switch1/3
  BL19/1 -> Logical Operator5/2
  Constant10/1 -> Switch5/3
  Saturation3/1 -> Rate Transition6/1
  BL13/1 -> [Brk2_On]
  Step5/1 -> Switch5/2
  Step6/1 -> Switch6/2

== system P2PHVDCMMC/Subsystem ==
  From1 : From  Commented=on  GotoTag=P  TagVisibility=global
  From10 : From  Commented=on  GotoTag=Vdc_kV_rec  TagVisibility=global
  From11 : From  Commented=on  GotoTag=Q  TagVisibility=global
  From2 : From  Commented=on  GotoTag=P  TagVisibility=global
  From28 : From  Commented=on  GotoTag=Vdc_kV_inv  TagVisibility=global
  From3 : From  Commented=on  GotoTag=P_inv  TagVisibility=global
  From36 : From  Commented=on  GotoTag=P_inv  TagVisibility=global
  From37 : From  Commented=on  GotoTag=Q_inv  TagVisibility=global
  From4 : From  Commented=on  GotoTag=Vdc_kV_rec  TagVisibility=global
  From5 : From  Commented=on  GotoTag=P_dqn_inv  TagVisibility=global
  From6 : From  Commented=on  GotoTag=Vdc_kV_dqn_rec  TagVisibility=global
  From7 : From  Commented=on  GotoTag=P_dqn_rec  TagVisibility=global
  From8 : From  Commented=on  GotoTag=Vdc_kV_dqn_inv  TagVisibility=global
  From9 : From  Commented=on  GotoTag=Vdc_kV_inv  TagVisibility=global
  Mux{,1..3} (4 alike) : Mux  Commented=on  Inputs=2
  P (MW) : Display  Commented=on
      settings: Format=bank  Decimation=5000
  P (MW)1 : Display  Commented=on
      settings: Format=bank  Decimation=5000
  Q (Mvar) : Display  Commented=on
      settings: Format=bank  Decimation=5000
  Q (Mvar)1 : Display  Commented=on
      settings: Format=bank  Decimation=5000
  Scope1 : Scope  Commented=on  NumInputPorts=2
  Scope2 : Scope  Commented=on  NumInputPorts=2
  Vdc (kV) : Display  Commented=on
      settings: Format=bank  Decimation=5000
  Vdc (kV)1 : Display  Commented=on
      settings: Format=bank  Decimation=5000
  wires:
  From8/1 -> Mux1/1
  From9/1 -> Mux/1
  From1/1 -> Mux2/1
  From6/1 -> Mux1/2
  From28/1 -> Vdc (kV)1/1
  From4/1 -> Vdc (kV)/1
  From36/1 -> P (MW)1/1
  From2/1 -> P (MW)/1
  Mux3/1 -> Scope2/1
  Mux/1 -> Scope1/2
  From10/1 -> Mux/2
  Mux2/1 -> Scope1/1
  From37/1 -> Q (Mvar)1/1
  From3/1 -> Mux2/2
  From5/1 -> Mux3/1
  From7/1 -> Mux3/2
  Mux1/1 -> Scope2/2
  From11/1 -> Q (Mvar)/1

== system P2PHVDCMMC/Subsystem3 ==
  g : Inport
  swL1 : spsIdealSwitchLib/Ideal Switch  Ron=0.01  Lon=0  IC=0  Rs=1e6  Cs=inf  Measurements=off
  swL2 : spsIdealSwitchLib/Ideal Switch  Ron=0.01  Lon=0  IC=0  Rs=1e6  Cs=inf  Measurements=off
  swL3 : spsIdealSwitchLib/Ideal Switch  Ron=0.01  Lon=0  IC=0  Rs=1e6  Cs=inf  Measurements=off
  in1 : PMIOPort  Side=Left
  in2 : PMIOPort  Port=2  Side=Left
  in3 : PMIOPort  Port=3  Side=Left
  o1 : PMIOPort  Port=4  Side=Right
  o2 : PMIOPort  Port=5  Side=Right
  o3 : PMIOPort  Port=6  Side=Right
  wires:
  g/1 -> swL2/1, swL3/1, swL1/1
  connections:
  swL3/RConn1 -- o3/RConn1
  swL3/LConn1 -- in3/RConn1
  swL2/LConn1 -- in2/RConn1
  swL1/LConn1 -- in1/RConn1
  swL1/RConn1 -- o1/RConn1
  swL2/RConn1 -- o2/RConn1

== system P2PHVDCMMC/Subsystem4 ==
  ACinv : Subsystem
  ACrec : Subsystem
  Constant4 : Constant  Value=S.x0  SampleTime=-1
  Constant6 : Constant  Value="complex( [[ 0 Vnom_prim*sqrt(2/3); 0 0; 0 0] zeros(3,N+2)  ])"
  DQsym_SS1 : DQsym_Lib/DQsym_SS  Ad=S.A  Bd=S.B  Cd=S.C  Dd=S.D  swOnRes=1e-2*ones(1,3)  swOffRes=1e6*ones(1,3)  swType=ones(1,3)  dt=Ts_dqn  nrSWvec=3
      settings: SourceProductName=DQsym Library
  Delay One Step2 : Delay  DelayLength=1  SampleTime=2e-5
  Gain : Gain  Gain=[1;1;1]
  Mux_DQNc_Mat : DQsym_Lib/Mux_DQNc_Mat  nrInp=5
      settings: SourceProductName=DQsym Library
  Subsystem : Subsystem
  SwitchCurrents1 : Constant  Value=zeros(3,N+4)
  wires:
  Constant4/1 -> DQsym_SS1/3
  Mux_DQNc_Mat/1 -> Delay One Step2/1
  ACrec/1(Out2) -> Mux_DQNc_Mat/3
  ACinv/1(Out2) -> Mux_DQNc_Mat/2
  SwitchCurrents1/1 -> Mux_DQNc_Mat/1
  Constant6/1 -> Mux_DQNc_Mat/5, Mux_DQNc_Mat/4
  Delay One Step2/1 -> DQsym_SS1/2
  Gain/1 -> DQsym_SS1/1
  DQsym_SS1/1 -> Subsystem/1(In2)
  [Brk2_On] -> Gain/1

== system P2PHVDCMMC/oltage urce1 ==
  In1 : Inport
  Demux9 : Demux  Outputs=3
  Ground : spsGroundLib/Ground  LConnTagsString=a
  VSRC_a : spsControlledVoltageSourceLib/Controlled Voltage Source  Initialize=on  Source_Type=AC  Amplitude=0  Phase=0  Frequency=0  Measurements=None
  VSRC_b : spsControlledVoltageSourceLib/Controlled Voltage Source  Initialize=on  Source_Type=AC  Amplitude=0  Phase=0  Frequency=0  Measurements=None
  VSRC_c : spsControlledVoltageSourceLib/Controlled Voltage Source  Initialize=on  Source_Type=AC  Amplitude=0  Phase=0  Frequency=0  Measurements=None
  a : PMIOPort  Side=Right
  b : PMIOPort  Port=2  Side=Right
  c : PMIOPort  Port=3  Side=Right
  wires:
  Demux9/3 -> VSRC_c/1
  Demux9/2 -> VSRC_b/1
  Demux9/1 -> VSRC_a/1
  In1/1 -> Demux9/1
  connections:
  VSRC_a/RConn1 -- a/RConn1
  VSRC_b/RConn1 -- b/RConn1
  VSRC_c/RConn1 -- c/RConn1
  VSRC_c/LConn1 -- VSRC_a/LConn1 -- VSRC_b/LConn1 -- Ground/LConn1

== system P2PHVDCMMC/oltage urce2 ==
  In1 : Inport
  Demux9 : Demux  Outputs=3
  Ground : spsGroundLib/Ground  LConnTagsString=a
  VSRC_a : spsControlledVoltageSourceLib/Controlled Voltage Source  Initialize=on  Source_Type=AC  Amplitude=0  Phase=0  Frequency=0  Measurements=None
  VSRC_b : spsControlledVoltageSourceLib/Controlled Voltage Source  Initialize=on  Source_Type=AC  Amplitude=0  Phase=0  Frequency=0  Measurements=None
  VSRC_c : spsControlledVoltageSourceLib/Controlled Voltage Source  Initialize=on  Source_Type=AC  Amplitude=0  Phase=0  Frequency=0  Measurements=None
  a : PMIOPort  Side=Right
  b : PMIOPort  Port=2  Side=Right
  c : PMIOPort  Port=3  Side=Right
  wires:
  Demux9/3 -> VSRC_c/1
  Demux9/2 -> VSRC_b/1
  Demux9/1 -> VSRC_a/1
  In1/1 -> Demux9/1
  connections:
  VSRC_a/RConn1 -- a/RConn1
  VSRC_b/RConn1 -- b/RConn1
  VSRC_c/RConn1 -- c/RConn1
  VSRC_c/LConn1 -- VSRC_a/LConn1 -- VSRC_b/LConn1 -- Ground/LConn1

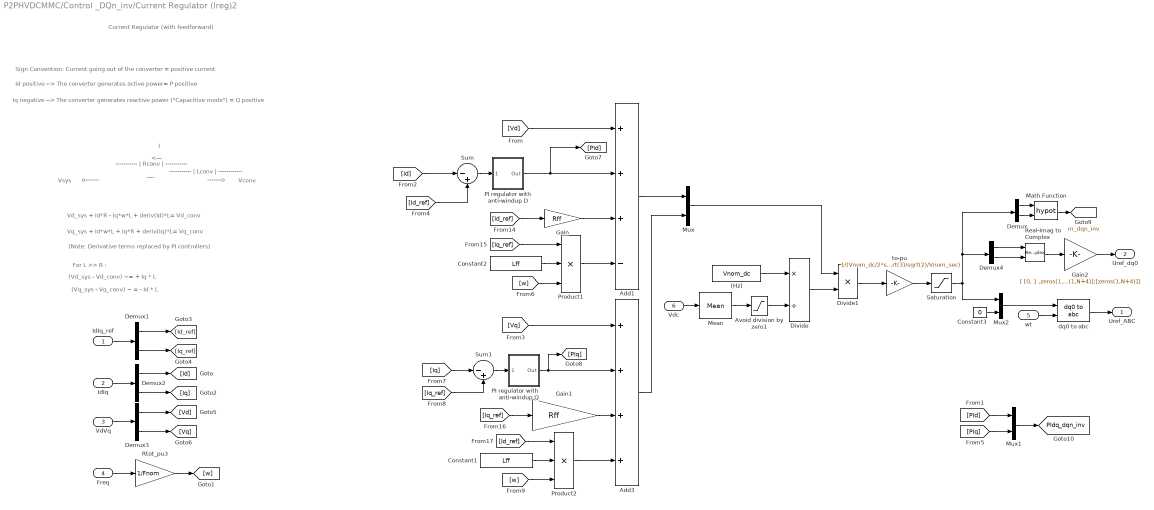
== system P2PHVDCMMC/Control _DQn_inv/Current Regulator (Ireg)2 ==
  note: -----------
      | | Lconv |
      | ------------
  note: <---
  note: -------o
  note: Vconv
  note: ----
  note: -----------
      | | Rconv |
      | -----------
  note: For L >> R :
  note: (Vq_sys - Vq_conv) ~ = - Id * L
  note: (Vd_sys - Vd_conv) ~= + Iq * L
  note: Id positive --> The converter generates active power= P positive
  note: Iq negative --> The converter generates reactive power ("Capacitive mode") = Q positive
  note: Sign Convention: Current going out of the converter = positive current
  note: Current Regulator
      | (with feedforward)
  note: Vq_sys + Id*w*L + Iq*R + deriv(Iq)*L= Vq_conv
  note: Vd_sys + Id*R - Iq*w*L + deriv(Id)*L= Vd_conv
  note: (Note: Derivative terms replaced by PI controllers)
  note: Vsys
  note: o-------
  note: I
  IdIq_ref : Inport  PortDimensions=2
  IdIq : Inport  Port=2  PortDimensions=2
  VdVq : Inport  Port=3  PortDimensions=2
  Freq : Inport  Port=4  PortDimensions=1
  wt : Inport  Port=5  PortDimensions=1
  Vdc : Inport  Port=6  PortDimensions=1
  " (Hz)" : Constant  Value=Vnom_dc  SampleTime=Ts
  Add1 : Sum  Inputs=+++-
  Add3 : Sum  Inputs=++++
  Avoid division by zero1 : Saturate  UpperLimit=Vnom_dc*1.25  LowerLimit=Vnom_dc*0.75
  Constant1 : Constant  Value=Lff  SampleTime=Ts_Control
  Constant2 : Constant  Value=Lff  SampleTime=Ts_Control
  Constant3 : Constant  Value=0  SampleTime=Ts
  Demux{,1..4} (5 alike) : Demux  Outputs=2
  Divide : Product  Inputs=*/
  Divide1 : Product  Inputs=**
  Gain : Gain  Gain=Rff
  Gain1 : Gain  Gain=Rff
  Gain2 : Gain  Gain=[ [0, 1 ,zeros(1,N+2)]; [zeros(1,N+4)];[zeros(1,N+4)]]
  Math Function : Math  Operator=hypot  SignedPower=on
  Mean : spsMeanLib/Mean  Freq=Fnom/3  Vinit=Vnom_dc  Ts=Ts
  Mux : Mux  Inputs=2
  Mux1 : Mux  Inputs=2
  Mux2 : Mux  Inputs=[2 1]
  PI regulator with anti-windup D : Subsystem  DialogController=POWERSYS.PowerSysDialog  mask(Discrete PI Controller){Kp=Kp_Ireg, Ki=Ki_Ireg, Par_Limits=Limits_Ireg, Init=0, Ts=Ts}
      mask prompts: Kp "Proportional gain (Kp):"; Ki "Integral gain (Ki):"; Par_Limits "Output limits: [ Upper   Lower ]"; Init "Output initial value:"; Ts "Sample time:"
      mask help: This block implements a discrete PI controller.
      mask init:
      | UpperLimit=Par_Limits(1);
      | LowerLimit=Par_Limits(2);
      | power_initmask();
      mask Help: This block is part of a subset of blocks in the Extras library that does not have documentation associated with it, other than the block mask description.
      mask Display: disp('PI');
  PI regulator with anti-windup Q : Subsystem  DialogController=POWERSYS.PowerSysDialog  mask(Discrete PI Controller){Kp=Kp_Ireg, Ki=Ki_Ireg, Par_Limits=Limits_Ireg, Init=0, Ts=Ts}
      mask prompts: Kp "Proportional gain (Kp):"; Ki "Integral gain (Ki):"; Par_Limits "Output limits: [ Upper   Lower ]"; Init "Output initial value:"; Ts "Sample time:"
      mask help: This block implements a discrete PI controller.
      mask init:
      | UpperLimit=Par_Limits(1);
      | LowerLimit=Par_Limits(2);
      | power_initmask();
      mask Help: This block is part of a subset of blocks in the Extras library that does not have documentation associated with it, other than the block mask description.
      mask Display: disp('PI');
  Product1 : Product  Inputs=3  RndMeth=Zero
  Product2 : Product  Inputs=3  RndMeth=Zero
  Real-Imag to Complex : RealImagToComplex
  Rtot_pu3 : Gain  Gain=1/Fnom  SaturateOnIntegerOverflow=on  OutDataTypeStr=Inherit: Same as input  ParamDataTypeStr=Inherit: Same as input
  Saturation : Saturate  UpperLimit=Limits_Ireg(1)  LowerLimit=Limits_Ireg(2)
  Sum : Sum  Inputs=|-+
  Sum1 : Sum  Inputs=|-+
  dq0 to abc : spsdq0toabcLib/dq0 to abc  Alignment=90 degrees behind phase A axis
  to-pu : Gain  Gain=1/(Vnom_dc/2*sqrt(3)/sqrt(2)/Vnom_sec)
  Uref_ABC : Outport
  Uref_dq0 : Outport  Port=2
  tag scope: PIdq_dqn_inv=global, m_dqn_inv=global
  wires:
  to-pu/1 -> Saturation/1
  Mux/1 -> Divide1/1
  dq0 to abc/1 -> Uref_ABC/1
  Divide/1 -> Divide1/2
  Mean/1 -> Avoid division by zero1/1
  Divide1/1 -> to-pu/1
  " (Hz)"/1 -> Divide/1
  Vdc/1 -> Mean/1
  Avoid division by zero1/1 -> Divide/2
  Mux1/1 -> [PIdq_dqn_inv]
  Constant3/1 -> Mux2/2
  Mux2/1 -> dq0 to abc/1
  PI regulator with anti-windup D/1(Out) -> [PId], Add1/2
  PI regulator with anti-windup Q/1(Out) -> [PIq], Add3/2
  [Vd] -> Add1/1
  Product1/1 -> Add1/4
  Gain/1 -> Add1/3
  Gain1/1 -> Add3/3
  Product2/1 -> Add3/4
  [Vq] -> Add3/1
  Demux2/1 -> [Id]
  IdIq/1 -> Demux2/1
  [Id_ref] -> Product2/1
  [Iq_ref] -> Gain1/1
  [Iq_ref] -> Product1/1
  [Id_ref] -> Gain/1
  [Id] -> Sum/1
  [Iq] -> Sum1/1
  Demux2/2 -> [Iq]
  [PIq] -> Mux1/2
  [PId] -> Mux1/1
  [w] -> Product1/3
  Constant2/1 -> Product1/2
  [w] -> Product2/3
  Constant1/1 -> Product2/2
  [Iq_ref] -> Sum1/2
  Sum1/1 -> PI regulator with anti-windup Q/1(Error)
  [Id_ref] -> Sum/2
  Sum/1 -> PI regulator with anti-windup D/1(Error)
  VdVq/1 -> Demux3/1
  Demux3/2 -> [Vq]
  Demux3/1 -> [Vd]
  IdIq_ref/1 -> Demux1/1
  Demux1/2 -> [Iq_ref]
  Demux1/1 -> [Id_ref]
  Rtot_pu3/1 -> [w]
  Freq/1 -> Rtot_pu3/1
  Add1/1 -> Mux/1
  Add3/1 -> Mux/2
  wt/1 -> dq0 to abc/2
  Demux4/2 -> Real-Imag to Complex/2
  Demux4/1 -> Real-Imag to Complex/1
  Real-Imag to Complex/1 -> Gain2/1
  Gain2/1 -> Uref_dq0/1
  Math Function/1 -> [m_dqn_inv]
  Demux/1 -> Math Function/1
  Demux/2 -> Math Function/2
  Saturation/1 -> Demux/1, Demux4/1, Mux2/1

== system P2PHVDCMMC/Control _DQn_inv/PLL, Measurements and Transformation1 ==
  note: Q positive = Converter generates reactive power (Capacitive Mode)
  note: P positive = Converter generates active power (Inverter Mode)
  note: Q (pu) = Vq*Id - Vd*Iq
  note: P (pu) = Vd*Id + Vq*Iq
  Vdq : Inport
  Idq : Inport  Port=2
  Add : Sum  Inputs=1
  Constant1 : Constant  Commented=on  Value=0.0004583
  Demux : Demux  Outputs=2
  Discrete Mean value : powerlib_extras/Discrete Measurements/Discrete  Mean value  Freq=Fnom  Vinit=0  Ts=Ts
  Discrete Mean value1 : powerlib_extras/Discrete Measurements/Discrete  Mean value  Freq=Fnom  Vinit=0  Ts=Ts
  From1 : From  Commented=on  TagVisibility=global
  I->pu2 : Gain  Gain=sqrt(3)*Vnom_sec/sqrt(2)/Pnom  SaturateOnIntegerOverflow=on  OutDataTypeStr=Inherit: Same as input  ParamDataTypeStr=Inherit: Same as input
  MATLAB Function : MATLAB Function  TreatAsAtomicUnit=on
  MATLAB Function1 : MATLAB Function  TreatAsAtomicUnit=on
  MATLAB Function2 : MATLAB Function  Commented=on  TreatAsAtomicUnit=on
  Mux : Mux  Inputs=2
  Mux1 : Mux  Inputs=2
  PLL (3ph) : Subsystem  Commented=on  AncestorBlock=|  DialogController=POWERSYS.PowerSysDialog  LoadFcn=sps_rtmsupport('LoadFcn', gcbh);  StartFcn=sps_rtmsupport('StartFcn', gcbh);  StopFcn=sps_rtmsupport('StopFcn', gcbh);  mask(PLL (3ph)){Fmin=0.9*Fnom, Par_Init=[0, Fnom], ParK=[180, 3200, 1], TcD=1e-4, MaxRateChangeFreq=12, FilterCutOffFreq=25, Ts=Ts, AGC=on}
      | spsPLL3phLib/PLL
      | (3ph)
      mask prompts: Fmin "Minimum frequency (Hz):"; Par_Init "Initial inputs [ Phase (degrees), Frequency (Hz) ]:"; ParK "Regulator gains [ Kp, Ki, Kd ]:"; TcD "Time constant for derivative action (s):"; MaxRateChangeFreq "Maximum rate of change of frequency (Hz/s):"; FilterCutOffFreq "Filter cut-off frequency for frequency measurement (Hz):"; Ts "Sample time:"; AGC "Enable automatic gain control"
      mask help:
      | This Phase Locked Loop (PLL) system can be used  to synchronize on a set of variable frequency, three-phase sinusoidal signals. If the Automatic Gain Control is enabled, the input (phase error) of the PLL regulator is scaled according to the input signals magnitude.
      |
      | For optimal performance, set regulator gains [ Kp Ki  Kd ] = [ 180  3200  1 ] and check the Enable Automatic Gain Control parameter.
      |
      | Input : Vector containing the normalized three-phase signals [Va Vb Vc]
      | Output 1:  Measured frequency (Hz) = w/(2pi)
      | Output 2:  Ramp w.t varying between  0 and 2*pi, synchronized on zero crossings of the fundamental (positive-sequence) of phase A.
      mask init:
      | block=gcb;
      | [WantBlockChoice,Ts,sps] = powericon('PLL3phInit',block,Fmin,Par_Init,ParK,TcD, MaxRateChangeFreq, FilterCutOffFreq, AGC,Ts);
      | powericon('SetInternalModels','set',block,WantBlockChoice);
      settings: CopyFcn=sps_rtmsupport('CopyFcn', gcbh);  DeleteFcn=sps_rtmsupport('DeleteFcn', gcbh);  UndoDeleteFcn=sps_rtmsupport('UndoDeleteFcn', gcbh);  ModelCloseFcn=sps_rtmsupport('ModelCloseFcn', gcbh);  PreSaveFcn=sps_rtmsupport('PreSaveFcn', gcbh);  PostSaveFcn=sps_rtmsupport('PostSaveFcn', gcbh);  NameChangeFcn=sps_rtmsupport('NameChangeFcn', gcbh);  PreCopyFcn=sps_rtmsupport('PreCopyFcn', gcbh);  OpenFcn=sps_rtmsupport('OpenFcn', gcbh, [8]);  CloseFcn=sps_rtmsupport('CloseFcn', gcbh);  PreDeleteFcn=sps_rtmsupport('PreDeleteFcn', gcbh);
      mask Help: helpview(psbhelp);
  PLL (3ph)2 : Subsystem  AncestorBlock=|  DialogController=POWERSYS.PowerSysDialog  LoadFcn=sps_rtmsupport('LoadFcn', gcbh);  StartFcn=sps_rtmsupport('StartFcn', gcbh);  StopFcn=sps_rtmsupport('StopFcn', gcbh);  mask(PLL (3ph)){Fmin=0.9*Fnom, Par_Init=[0, Fnom], ParK=[180, 3200, 1], TcD=1e-4, MaxRateChangeFreq=12, FilterCutOffFreq=25, Ts=Ts, AGC=on}
      | spsPLL3phLib/PLL
      | (3ph)
      mask prompts: Fmin "Minimum frequency (Hz):"; Par_Init "Initial inputs [ Phase (degrees), Frequency (Hz) ]:"; ParK "Regulator gains [ Kp, Ki, Kd ]:"; TcD "Time constant for derivative action (s):"; MaxRateChangeFreq "Maximum rate of change of frequency (Hz/s):"; FilterCutOffFreq "Filter cut-off frequency for frequency measurement (Hz):"; Ts "Sample time:"; AGC "Enable automatic gain control"
      mask help:
      | This Phase Locked Loop (PLL) system can be used  to synchronize on a set of variable frequency, three-phase sinusoidal signals. If the Automatic Gain Control is enabled, the input (phase error) of the PLL regulator is scaled according to the input signals magnitude.
      |
      | For optimal performance, set regulator gains [ Kp Ki  Kd ] = [ 180  3200  1 ] and check the Enable Automatic Gain Control parameter.
      |
      | Input : Vector containing the normalized three-phase signals [Va Vb Vc]
      | Output 1:  Measured frequency (Hz) = w/(2pi)
      | Output 2:  Ramp w.t varying between  0 and 2*pi, synchronized on zero crossings of the fundamental (positive-sequence) of phase A.
      mask init:
      | block=gcb;
      | [WantBlockChoice,Ts,sps] = powericon('PLL3phInit',block,Fmin,Par_Init,ParK,TcD, MaxRateChangeFreq, FilterCutOffFreq, AGC,Ts);
      | powericon('SetInternalModels','set',block,WantBlockChoice);
      settings: CopyFcn=sps_rtmsupport('CopyFcn', gcbh);  DeleteFcn=sps_rtmsupport('DeleteFcn', gcbh);  UndoDeleteFcn=sps_rtmsupport('UndoDeleteFcn', gcbh);  ModelCloseFcn=sps_rtmsupport('ModelCloseFcn', gcbh);  PreSaveFcn=sps_rtmsupport('PreSaveFcn', gcbh);  PostSaveFcn=sps_rtmsupport('PostSaveFcn', gcbh);  NameChangeFcn=sps_rtmsupport('NameChangeFcn', gcbh);  PreCopyFcn=sps_rtmsupport('PreCopyFcn', gcbh);  OpenFcn=sps_rtmsupport('OpenFcn', gcbh, [8]);  CloseFcn=sps_rtmsupport('CloseFcn', gcbh);  PreDeleteFcn=sps_rtmsupport('PreDeleteFcn', gcbh);
      mask Help: helpview(psbhelp);
  Product : Product  RndMeth=Zero
  Product1 : Product  RndMeth=Zero
  Rate Transition3 : RateTransition  OutPortSampleTime=Ts_Control
  Second-Order Filter2 : spsSecondOrderFilterLib/Second-Order Filter  FilterType=Lowpass  Fo=Fn_filter  Zeta=Zeta_filter  Ts=Ts  Initialize=off  Vac_Init="[0,  0,  60]"  Vdc_Init=0  PlotResponse=off  FreqRange=[0, 500, 1]
  Second-Order Filter3 : spsSecondOrderFilterLib/Second-Order Filter  FilterType=Lowpass  Fo=Fn_filter  Zeta=Zeta_filter  Ts=Ts  Initialize=off  Vac_Init="[0,  0,  60]"  Vdc_Init=0  PlotResponse=off  FreqRange=[0, 500, 1]
  Selector3 : Selector  InputPortWidth=2  IndexOptions=Index vector (dialog)  Indices=[2 1]  OutputSizes=1
  Subtract : Sum  Inputs=+-
  Sum : Sum  Inputs=|+-
  V->pu1 : Gain  Gain=1/(Vnom_sec/sqrt(3)*sqrt(2))  SaturateOnIntegerOverflow=on  OutDataTypeStr=Inherit: Same as input  ParamDataTypeStr=Inherit: Same as input
  Freq : Outport
  wt : Outport  Port=2
  VdVq : Outport  Port=3
  IdIq : Outport  Port=4
  P : Outport  Port=5
  Q : Outport  Port=6
  wires:
  Idq/1 -> I->pu2/1
  PLL (3ph)2/2(wt) -> Sum/1, wt/1
  Vdq/1 -> V->pu1/1
  PLL (3ph)2/1(Freq) -> Freq/1
  Subtract/1 -> Discrete Mean value1/1
  Add/1 -> Discrete Mean value/1
  Demux/2 -> Subtract/2
  Demux/1 -> Subtract/1
  Product1/1 -> Demux/1
  Product/1 -> Add/1
  Discrete Mean value/1 -> P/1
  Discrete Mean value1/1 -> Q/1
  Selector3/1 -> Product1/1
  Second-Order Filter2/1 -> Selector3/1, Product/1, VdVq/1
  Second-Order Filter3/1 -> Product/2, Product1/2, IdIq/1
  MATLAB Function/1(d) -> Mux/1
  Sum/1 -> MATLAB Function1/2(wt), MATLAB Function/2(wt)
  MATLAB Function/2(q) -> Mux/2
  Mux/1 -> Second-Order Filter2/1
  V->pu1/1 -> PLL (3ph)2/1(DQ), MATLAB Function/1(DQ)
  Mux1/1 -> Second-Order Filter3/1
  MATLAB Function1/1(d) -> Mux1/1
  I->pu2/1 -> MATLAB Function1/1(DQ)
  MATLAB Function1/2(q) -> Mux1/2
  Rate Transition3/1 -> Sum/2
  [wt0] -> Rate Transition3/1

== system P2PHVDCMMC/Control _DQn_inv/Reactive Power Regulator ==
  note: P (pu) = Vd*Id + Vq*Iq (Zero-sequence is not taken into account)
  note: Q (pu) = Vq*Id - Vd*Iq (valid only for balanced & harmonics-free values)
  note: If PLL sync on Vprim --> Vq=0 --> Id = P/Vd et Iq = -1.0 * Q/Vd
  note: Reactive Power Regulator
  VdVq_mes : Inport  PortDimensions=2
  Qmes : Inport  Port=2  PortDimensions=1
  On : Inport  Port=3  PortDimensions=1
  Qref : Inport  Port=4  PortDimensions=1
  Add2 : Sum
  Discrete Mean value1 : powerlib_extras/Discrete Measurements/Discrete  Mean value  Freq=Fnom  Vinit=0  Ts=Ts
  Discrete-Time Integrator : DiscreteIntegrator  SampleTime=Ts  LimitOutput=on  UpperSaturationLimit=Limits_Qreg(1)  LowerSaturationLimit=Limits_Qreg(2)  ICPrevOutput=DiscIntNeverNeededParam  ICPrevScaledInput=DiscIntNeverNeededParam
  Divide : Product  Inputs=*/
  Product : Product  RndMeth=Zero
  Product1 : Product  RndMeth=Zero
  Rtot_pu1 : Gain  Gain=-1  SaturateOnIntegerOverflow=on  OutDataTypeStr=Inherit: Same as input  ParamDataTypeStr=Inherit: Same as input
  Rtot_pu2 : Gain  Gain=-1  SaturateOnIntegerOverflow=on  OutDataTypeStr=Inherit: Same as input  ParamDataTypeStr=Inherit: Same as input
  Saturation : Saturate  UpperLimit=Limits_Qreg(1)  LowerLimit=Limits_Qreg(2)
  Saturation1 : Saturate  UpperLimit=2  LowerLimit=1e-6
  Saturation2 : Saturate  UpperLimit=Limits_Qreg(1)  LowerLimit=Limits_Qreg(2)
  Selector : Selector  InputPortWidth=2  IndexOptions=Index vector (dialog)  Indices=[1]  OutputSizes=1
  Sum : Sum  Inputs=|-+
  Sum6 : Sum  InputSameDT=on  SaturateOnIntegerOverflow=on  SampleTime=Ts  OutDataTypeStr=Inherit: Same as first input
  Switch1 : Switch  Criteria=u2 ~= 0  Threshold=0.5  OutDataTypeStr=double  SaturateOnIntegerOverflow=off  InputSameDT=off
  VdcNom_SM : Constant  Value=Kp_Qreg
  VdcNom_SM1 : Constant  Value=Ki_Qreg
  Zero-Order Hold : ZeroOrderHold  SampleTime=Ts
  Iq_ref : Outport
  wires:
  Qref/1 -> Sum/2, Switch1/3, Divide/1
  Qmes/1 -> Sum/1
  VdVq_mes/1 -> Selector/1
  Selector/1 -> Discrete Mean value1/1
  Divide/1 -> Rtot_pu2/1
  Saturation1/1 -> Divide/2
  Discrete Mean value1/1 -> Saturation1/1
  Zero-Order Hold/1 -> Sum6/1
  Discrete-Time Integrator/1 -> Sum6/2
  VdcNom_SM1/1 -> Product/1
  VdcNom_SM/1 -> Product1/1
  Product1/1 -> Zero-Order Hold/1
  Product/1 -> Discrete-Time Integrator/1
  Add2/1 -> Saturation/1
  On/1 -> Switch1/2
  Sum/1 -> Switch1/1
  Switch1/1 -> Product/2, Product1/2
  Sum6/1 -> Saturation2/1
  Rtot_pu1/1 -> Add2/1
  Rtot_pu2/1 -> Add2/2
  Saturation/1 -> Iq_ref/1
  Saturation2/1 -> Rtot_pu1/1
